simulink model "control_01"  (R2019b)
settings: Solver=VariableStepAuto  StartTime=0.0  StopTime=100  RelTol=1e-3
InitFcn:
  | A=1.2
  | rho=1
  | c = 0.4
  | b = 10
  | m = 1250
settings Model: Creator=IGG2BP  LastModifiedBy=IGG2BP

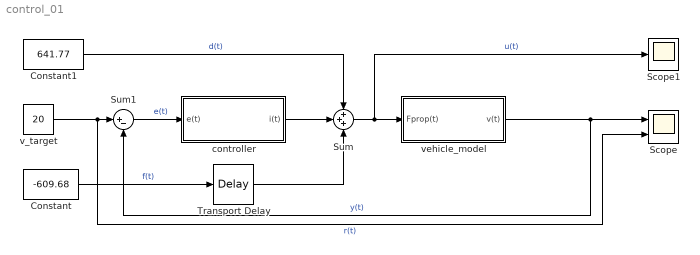
== system control_01 ==
  Constant : Constant  Value=-609.68
  Constant1 : Constant  Value=641.77
  Scope : Scope  NumInputPorts=2
  Scope1 : Scope
  Sum : Sum  Inputs=+++
  Sum1 : Sum  Inputs=|+-
  Transport Delay : TransportDelay  DelayTime=0.5
  controller : Subsystem
  v_target : Constant  Value=20
  vehicle_model : Subsystem
  wires:
  Sum/1 -> Scope1/1, vehicle_model/1(Fprop(t))  "u(t)"
  Sum1/1 -> controller/1(e(t))  "e(t)"
  vehicle_model/1(v(t)) -> Scope/1, Sum1/2  "y(t)"
  v_target/1 -> Scope/2, Sum1/1  "r(t)"
  Constant/1 -> Transport Delay/1  "f(t)"
  Constant1/1 -> Sum/1  "d(t)"
  controller/1(i(t)) -> Sum/2
  Transport Delay/1 -> Sum/3

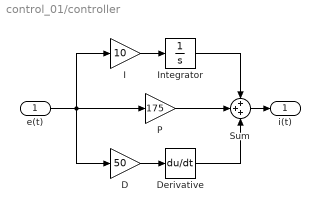
== system control_01/controller ==
  e(t) : Inport
  D : Gain  Gain=50
  Derivative : Derivative  CoefficientInTFapproximation=0
  I : Gain  Gain=10
  Integrator : Integrator
  P : Gain  Gain=175
  Sum : Sum  Inputs=+++
  i(t) : Outport
  wires:
  e(t)/1 -> D/1, I/1, P/1
  I/1 -> Integrator/1
  Integrator/1 -> Sum/1
  P/1 -> Sum/2
  Sum/1 -> i(t)/1
  D/1 -> Derivative/1
  Derivative/1 -> Sum/3

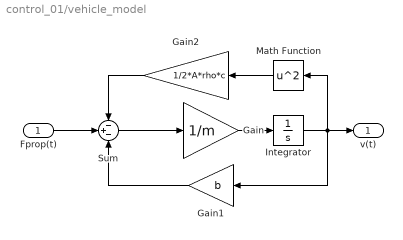
== system control_01/vehicle_model ==
  Fprop(t) : Inport
  Gain : Gain  Gain=1/m
  Gain1 : Gain  Gain=b
  Gain2 : Gain  Gain=1/2*A*rho*c
  Integrator : Integrator  InitialCondition=15
  Math Function : Math  Operator=square  SignedPower=off  SaturateOnIntegerOverflow=on
  Sum : Sum  Inputs=-+-
  v(t) : Outport
  wires:
  Integrator/1 -> Math Function/1, Gain1/1, v(t)/1
  Gain/1 -> Integrator/1
  Gain1/1 -> Sum/3
  Sum/1 -> Gain/1
  Fprop(t)/1 -> Sum/2
  Math Function/1 -> Gain2/1
  Gain2/1 -> Sum/1
